simulink model "Model_Automatique_BF_PI"  (R2020a)
settings: Solver=VariableStepAuto  StartTime=0.0  StopTime=tfinal  RelTol=1e-6
values from neighbouring files (symbols this model uses):
  Kc = 0.10416    [Simulation_Trottinette.m]    (also in Simulation_Trottinette_BF.m)
  Kh = 2*Ubat    (= 48)    [Simulation_Trottinette.m]    (also in Simulation_Trottinette_BF.m)
  L = 2e-3    (= 0.002)    [Simulation_Trottinette.m]    (also in Simulation_Trottinette_BF.m)
  R = 1    [Simulation_Trottinette.m]    (also in Simulation_Trottinette_BF.m)
  tfinal = 10e-3    (= 0.01)    [Simulation_Trottinette.m]    (also in Simulation_Trottinette_BF.m)
  Yc = 0.5    [Simulation_Trottinette.m]    (also in Simulation_Trottinette_BF.m)
undefined symbols (not defined in the file or in its folder): den1, den2, Kfiltre, tau3, tau4
settings Model: Creator=mdescham  LastModifiedBy=mdescham

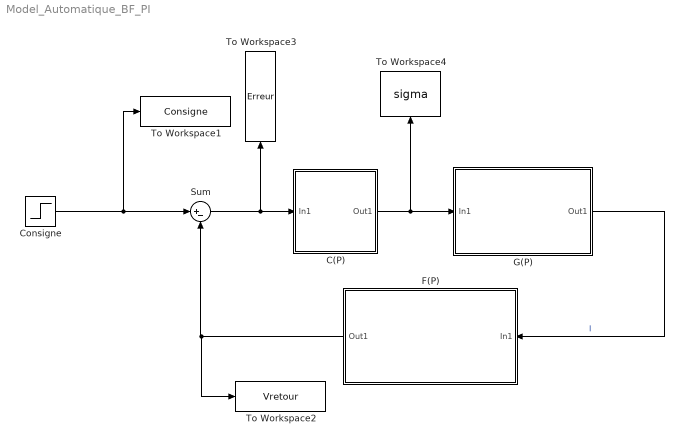
== system Model_Automatique_BF_PI ==
  C(P) : Subsystem
  Consigne : Step  Time=tfinal/8  After=Yc  SampleTime=0
  F(P) : Subsystem
  G(P) : Subsystem
  Sum : Sum  Inputs=|+-
  To Workspace1 : ToWorkspace  VariableName=Consigne  SaveFormat=Timeseries  SampleTime=-1
  To Workspace2 : ToWorkspace  VariableName=Vretour  SaveFormat=Timeseries  SampleTime=-1
  To Workspace3 : ToWorkspace  VariableName=Erreur  SaveFormat=Timeseries  SampleTime=-1
  To Workspace4 : ToWorkspace  VariableName=sigma  SaveFormat=Timeseries  SampleTime=-1
  wires:
  C(P)/1(Out1) -> G(P)/1(In1), To Workspace4/1
  Consigne/1 -> Sum/1, To Workspace1/1
  G(P)/1(Out1) -> F(P)/1(In1)  "I"
  Sum/1 -> To Workspace3/1, C(P)/1(In1)
  F(P)/1(Out1) -> To Workspace2/1, Sum/2

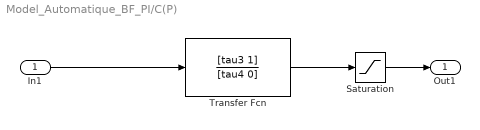
== system Model_Automatique_BF_PI/C(P) ==
  In1 : Inport
  Saturation : Saturate
  Transfer Fcn : TransferFcn  Numerator=[tau3 1]  Denominator=[tau4 0]
  Out1 : Outport
  wires:
  In1/1 -> Transfer Fcn/1
  Transfer Fcn/1 -> Saturation/1
  Saturation/1 -> Out1/1

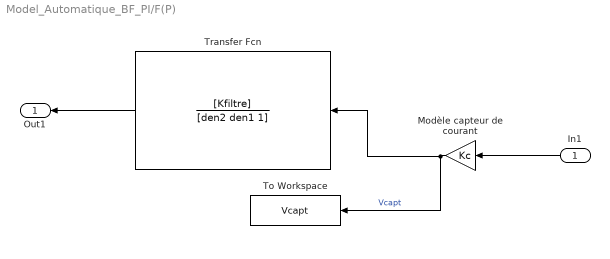
== system Model_Automatique_BF_PI/F(P) ==
  In1 : Inport
  Modèle capteur de courant : Gain  Gain=Kc
  To Workspace : ToWorkspace  VariableName=Vcapt  SaveFormat=Timeseries  SampleTime=-1
  Transfer Fcn : TransferFcn  Numerator=[Kfiltre]  Denominator=[den2 den1 1]
  Out1 : Outport
  wires:
  Modèle capteur de courant/1 -> To Workspace/1, Transfer Fcn/1  "Vcapt"
  Transfer Fcn/1 -> Out1/1
  In1/1 -> Modèle capteur de courant/1

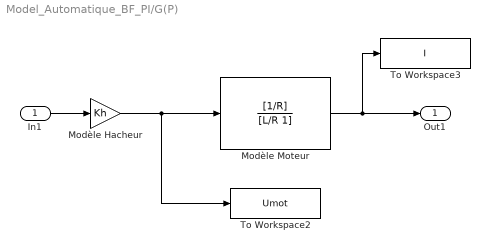
== system Model_Automatique_BF_PI/G(P) ==
  In1 : Inport
  Modèle Hacheur : Gain  Gain=Kh
  Modèle Moteur : TransferFcn  Numerator=[1/R]  Denominator=[L/R 1]
  To Workspace2 : ToWorkspace  VariableName=Umot  SaveFormat=Timeseries  SampleTime=-1
  To Workspace3 : ToWorkspace  VariableName=I  SaveFormat=Timeseries  SampleTime=-1
  Out1 : Outport
  wires:
  Modèle Hacheur/1 -> To Workspace2/1, Modèle Moteur/1
  Modèle Moteur/1 -> Out1/1, To Workspace3/1
  In1/1 -> Modèle Hacheur/1
